simulink model "DIMR_ordinary"  (R2024b)
settings: Solver=daessc  StartTime=0.0  StopTime=60  RelTol=1e-3
values from neighbouring files (symbols this model uses):
  d_m0 = d_mn    (= 0)    [DIMR_main.m]
  d_m_cmd = 0.12787808985686    (= 0.127878089857)    [DIMR_main.m]
  dis_cmd = 0    [DIMR_main.m]
  jrk_cmd = 0.15    [DIMR_main.m]
  phi_cmd = 0*pi/180    (= 0)    [DIMR_main.m]
  ta = (vel_cmd-jrk_cmd*tt^2)/acc_cmd    (= 3.66666666667)    [DIMR_main.m]
  taz = z_vel_cmd/z_acc_cmd    (= 1.6)    [DIMR_main.m]
  tc = (x_cmd-2*(1/2*acc_cmd*ta^2+1/2*jrk_cmd*tt^2*ta+tt*vel_cmd))/vel_cmd    (= 10.6666666667)    [DIMR_main.m]
  tcz = (z_cmd-z_acc_cmd*taz^2)/z_vel_cmd    [DIMR_main.m]
  tcz2 = (z_cmd2-z_acc_cmd*taz^2)/z_vel_cmd    (= 0.9)    [DIMR_main.m]
  theta_f0 = -theta_p0    (= -0.024)    [DIMR_main.m]
  theta_f_cmd = 0.037940459    [DIMR_main.m]
  theta_p0 = theta_pn    (= 0.024)    [DIMR_main.m]
  theta_p_cmd = -0.037940459    [DIMR_main.m]
  ts = 15    [DIMR_main.m]
  ts2 = te+5    (= 39.3333333333)    [DIMR_main.m]
  tsz = 10    [DIMR_main.m]
  tsz2 = ts2    (= 39.3333333333)    [DIMR_main.m]
  tt = acc_cmd/jrk_cmd    (= 0.333333333333)    [DIMR_main.m]
  x_cmd = 3    [DIMR_main.m]
  z_0 = R_wo+L_bmy+L_my/2    [DIMR_main.m]
  z_acc_cmd = 0.05    [DIMR_main.m]
  z_cmd = 0.9-z_0    [DIMR_main.m]
  z_cmd2 = 0.9-0.7    (= 0.2)    [DIMR_main.m]
undefined symbols (not defined in the file or in its folder): Ac, Dc, DiscIntNeverNeededParam, dspblkCoreblockFVToolHelper, g, g_ext, g_fork, g_lift, g_reac, g_spado, g_yaw, gcbh, K_fd, K_fp, K_md, K_mp, K_pd, K_pp, K_wd, K_wi, K_wp, K_yd, K_yp, Kc, L_bg, L_bmx, L_bmy, L_bmz, L_bsx, L_bsy, L_bsz, L_by, L_ex, L_ey, L_ez, L_fg, L_fh, L_fx, L_fy, L_fz, L_lx, L_ly, L_lz, L_mg, L_mx, L_my, L_mz, L_wt, M_b, M_f, M_m, M_n11, M_n21, M_n22, M_n33, M_n44, Mc, N_f, N_w, omega_c ... (+10)
libraries: simulink x56, sm_lib x54, nesl_utility x12, slctrl_autotuning x1, slpidlib x1
(part 4 of 6)

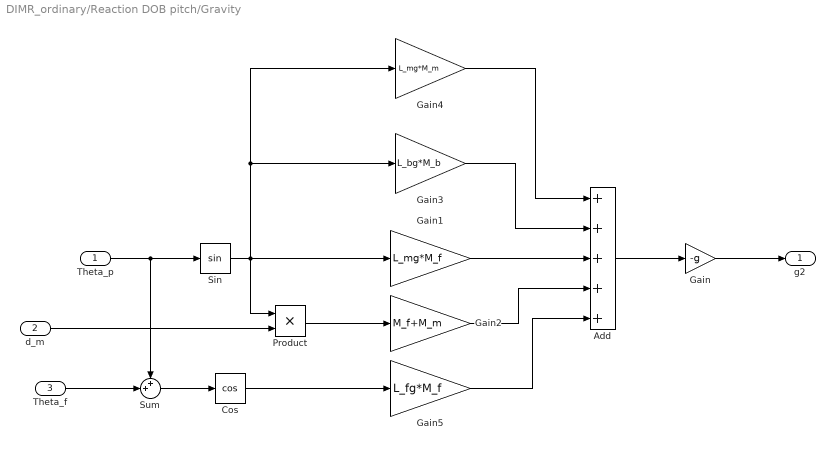
== system DIMR_ordinary/Reaction DOB pitch/Gravity ==
  Theta_p : Inport
  d_m : Inport  Port=2
  Theta_f : Inport  Port=3
  Add : Sum  Inputs=+++++
  Cos : Trigonometry  Operator=cos
  Gain : Gain  Gain=-g
  Gain1 : Gain  Gain=L_mg*M_f
  Gain2 : Gain  Gain=M_f+M_m
  Gain3 : Gain  Gain=L_bg*M_b
  Gain4 : Gain  Gain=L_mg*M_m
  Gain5 : Gain  Gain=L_fg*M_f
  Product : Product
  Sin : Trigonometry
  Sum : Sum  Inputs=++|
  g2 : Outport
  wires:
  Gain/1 -> g2/1
  Theta_p/1 -> Sin/1, Sum/1
  Sin/1 -> Gain4/1, Gain3/1, Product/1, Gain1/1
  d_m/1 -> Product/2
  Product/1 -> Gain2/1
  Theta_f/1 -> Sum/2
  Sum/1 -> Cos/1
  Cos/1 -> Gain5/1
  Add/1 -> Gain/1
  Gain4/1 -> Add/1
  Gain3/1 -> Add/2
  Gain1/1 -> Add/3
  Gain2/1 -> Add/4
  Gain5/1 -> Add/5

== matlab function DIMR_ordinary/IK1 ==
  data: dz input; tau input; z input; ik_theta1 output; ik_delta2 output; ik_dtheta1 output; ik_ddelta2 output; ik_lt output
function [ik_theta1,ik_delta2,ik_dtheta1,ik_ddelta2,ik_lt] = IK1(dz,tau,z)
%#codegen

%    This function was generated by the Symbolic Math Toolbox version 24.2.
%    15-Apr-2025 18:25:07

% dz = complex(dz);  % if required to enforce complex operations
% tau = complex(tau);  % if required to enforce complex operations
% z = complex(z);  % if required to enforce complex operations
t0 = roots([1.0,(tau.*8.44424930131968e+16-z.*6.07271847679102e+19-tau.*z.*1.125899906842624e+18+2.195986091984785e+19)./(tau.*1.238489897526886e+17+9.351986454258171e+17),0.0,((tau.*-8.44424930131968e+16+z.*6.07271847679102e+19+tau.*z.*1.125899906842624e+18+1.285078320466132e+19).*(-1.0./4.4e+2))./(tau.*2.81474976710656e+14+2.125451466876857e+15),-1.0]);
t2 = real(t0(4));
t3 = atan2(t2,1);
t4 = t2.^2;
t5 = t2.^3;
t6 = tau.^2;
t7 = tau.^3;
t9 = tau.^5;
t11 = z.^2;
t12 = z.^3;
t14 = z.^5;
t19 = tau.*1.40737488355328e+14;
t20 = tau.*5.319877059831398e+17;
t21 = t2.*tau.*1.238489897526886e+17;
t22 = t2.*9.351986454258171e+17;
t23 = tau.*z.*1.125899906842624e+18;
t24 = z.*6.07271847679102e+19;
t35 = tau.*4.635073695354219e-1;
t57 = tau.*5.743900035854321e+113;
t66 = tau.*z.*7.990597029423474e+114;
t74 = z.*1.447317376015955e+116;
t8 = t6.^2;
t10 = t6.^3;
t13 = t11.^2;
t15 = t11.^3;
t16 = t3.*2.0;
ik_theta1 = t16;
if nargout > 1
    t25 = -t23;
    t26 = -t24;
    t27 = t4.*tau.*8.44424930131968e+16;
    t28 = t5.*tau.*1.238489897526886e+17;
    t29 = t5.*9.351986454258171e+17;
    t30 = t4.*2.195986091984785e+19;
    t33 = t4.*tau.*z.*-1.125899906842624e+18;
    t34 = t4.*z.*-6.07271847679102e+19;
    t36 = t19+7.590898095988775e+15;
    t38 = t35+7.0./2.0;
    t39 = t35+6.81e+2./1.0e+1;
    t42 = t9.*2.386050182016105e+106;
    t46 = t9.*z.*4.211088297564564e+107;
    t51 = t7.*2.507343178421252e+110;
    t52 = t9.*t11.*4.593987726794744e+108;
    t58 = t9.*t12.*2.604615627247899e+109;
    t60 = t6.*2.999842761429269e+112;
    t61 = t7.*z.*9.409126505705104e+111;
    t65 = t9.*t14.*2.966510080312107e+110;
    t72 = -t66;
    t73 = t6.*z.*3.660741181676567e+113;
    t75 = t7.*t11.*6.407841099867219e+112;
    t76 = t7.*t12.*3.958710038416369e+112;
    t81 = -t74;
    t86 = t11.*tau.*3.585353509436109e+115;
    t87 = t6.*t11.*2.09113906624741e+114;
    t88 = t6.*t12.*3.785302651403782e+114;
    t90 = t7.*t14.*2.876678343420641e+114;
    t92 = t11.*7.09032593341523e+116;
    t93 = t12.*tau.*2.133985804221304e+116;
    t95 = t12.*3.242008287042286e+117;
    t98 = t14.*2.256895254686051e+118;
    t101 = t14.*tau.*2.510610198759619e+117;
    t102 = t6.*t14.*1.163686329155874e+116;
    t17 = cos(t16);
    t18 = sin(t16);
    t37 = 1.0./t36;
    t40 = 1.0./t39.^2;
    t41 = t10.*3.212055390272792e+104;
    t43 = t10.*z.*2.675474179773727e+105;
    t44 = t8.*2.477746168797788e+107;
    t47 = t10.*t11.*2.526492816377412e+106;
    t48 = -t46;
    t49 = t10.*t12.*1.059207781794524e+107;
    t50 = t10.*t13.*4.676525342669896e+107;
    t54 = t10.*t14.*9.166661893505187e+107;
    t55 = t10.*t15.*2.037035976334486e+108;
    t56 = t8.*z.*9.736596647488009e+109;
    t63 = -t58;
    t64 = t9.*t13.*1.239018969121646e+110;
    t67 = -t61;
    t68 = t8.*t11.*7.882227863274746e+110;
    t69 = t8.*t12.*2.154890938178742e+111;
    t70 = -t65;
    t71 = t9.*t15.*6.592244622915794e+110;
    t78 = t8.*t13.*1.21830758387732e+112;
    t79 = t8.*t14.*4.00008483587525e+112;
    t80 = -t73;
    t82 = -t76;
    t83 = t7.*t13.*4.915417942081258e+113;
    t85 = t8.*t15.*8.88907741305611e+112;
    t89 = t6.*t13.*1.928403609769147e+114;
    t91 = t7.*t15.*6.392618540934758e+114;
    t94 = t13.*tau.*3.97502326562149e+116;
    t96 = -t90;
    t97 = t13.*7.985575221783389e+117;
    t99 = t15.*5.015322788191225e+118;
    t103 = t6.*t15.*2.585969620346386e+116;
    t105 = -t98;
    t106 = -t101;
    t107 = t15.*tau.*5.579133775021375e+117;
    t108 = -t102;
    t109 = t20+t21+t22+t25+t26+t27+t28+t29+t30+t33+t34+2.869359480283757e+19;
    t45 = -t43;
    t53 = -t49;
    t59 = -t54;
    t62 = -t56;
    t77 = -t69;
    t84 = -t79;
    t100 = -t94;
    t104 = -t97;
    t110 = (t37.*t109)./8.0e+3;
    ik_delta2 = -t110;
end
if nargout > 2
    t111 = t110-1.59e+2./4.0e+2;
    t112 = t41+t42+t44+t45+t47+t48+t50+t51+t52+t53+t55+t57+t59+t60+t62+t63+t64+t67+t68+t70+t71+t72+t75+t77+t78+t80+t81+t82+t83+t84+t85+t86+t87+t88+t89+t91+t92+t93+t95+t96+t99+t100+t103+t104+t105+t106+t107+t108-2.105477541297374e+115;
    t113 = 1.0./t112;
    et1 = t2.*-1.753894605876528e+96+t4.*1.009464978528226e+96;
    et2 = t5.*4.619988807297373e+94-t6.*2.554852704393891e+92;
    et3 = t7.*-7.8111064788263e+89-t8.*1.00794759003273e+89;
    et4 = t9.*1.814387972119789e+86+t11.*6.245124509053326e+96;
    et5 = t12.*-3.331857083120826e+97;
    et6 = t13.*3.815554989087441e+97-tau.*5.24829876676123e+94;
    et7 = z.*1.399328629129073e+96-t2.*t6.*1.075720720231548e+91;
    et8 = t2.*t7.*-1.388092428471541e+90+t2.*t8.*7.128076116355089e+88;
    et9 = t4.*t6.*1.722969069981006e+93+t2.*t9.*1.361707336651519e+86;
    et10 = t4.*t7.*-1.973567476521639e+90+t5.*t6.*9.078257330103773e+92;
    et11 = t4.*t8.*1.151036106739522e+89+t5.*t7.*6.111449310419045e+90;
    et12 = t2.*t11.*5.875732481208788e+97+t4.*t9.*1.343184695804828e+87;
    et13 = t5.*t8.*-2.551325158332646e+88-t2.*t12.*1.782863198738202e+97;
    et14 = t5.*t9.*5.322204718218049e+86-t2.*t13.*5.464130766461227e+98;
    et15 = t4.*t11.*4.415911382468272e+97;
    et16 = t2.*t14.*8.258777032656798e+98;
    et17 = t4.*t12.*-8.469349253727501e+97;
    et18 = t5.*t11.*9.380726613532944e+95;
    et19 = t4.*t13.*6.359258315145734e+97;
    et20 = t5.*t12.*-1.175190936638932e+96+t6.*t11.*5.907708747848193e+94;
    et21 = t6.*t12.*-3.196898258866477e+95+t7.*t11.*1.247609721739556e+93;
    et22 = t6.*t13.*4.534279766579717e+95-t7.*t12.*6.544610701214467e+93;
    et23 = t8.*t11.*1.242487226117768e+91+t7.*t13.*1.139418916775499e+94;
    et24 = t8.*t12.*-5.845583673798496e+91+t9.*t11.*4.904790067467224e+88;
    et25 = t8.*t13.*1.333203858988986e+92-t9.*t12.*1.791158880389735e+89;
    et26 = t9.*t13.*5.970529601299116e+89+tau.*t2.*1.323988270291723e+93;
    et27 = t4.*tau.*1.468522013529346e+95+t5.*tau.*1.261219729665987e+94;
    et28 = t11.*tau.*1.207196483550789e+96;
    et29 = t12.*tau.*-6.477833809662083e+96;
    et30 = t13.*tau.*7.882625873837409e+96;
    et31 = z.*t2.*-1.890970205684437e+96;
    et32 = t4.*z.*-1.069218722198518e+97;
    et33 = t5.*z.*-3.150739272925472e+95+t6.*z.*2.668557352126731e+93;
    et34 = t7.*z.*4.092978643690637e+91+t8.*z.*6.846342443053817e+89;
    et35 = t9.*z.*-5.342131360762384e+87+tau.*z.*2.034429880145039e+95;
    et36 = t2.*t6.*t11.*3.834597488658114e+94+t2.*t6.*t12.*1.79267290146031e+95;
    et37 = t2.*t7.*t11.*3.241447763154754e+92-t2.*t6.*t13.*1.552786419763549e+96;
    et38 = t2.*t7.*t12.*4.397794916127146e+93+t2.*t8.*t11.*6.696326945473049e+89;
    et39 = t4.*t6.*t11.*2.979273638991897e+95;
    et40 = t2.*t6.*t14.*2.838892916716577e+96;
    et41 = t2.*t7.*t13.*-2.577198424443163e+94+t2.*t8.*t12.*4.358240682659937e+91;
    et42 = t2.*t9.*t11.*-1.748415316198616e+88-t4.*t6.*t12.*7.776982869967544e+95;
    et43 = t4.*t7.*t11.*4.360273950273173e+93+t5.*t6.*t11.*2.746751487155486e+94;
    et44 = t2.*t7.*t14.*5.263391152880169e+94-t2.*t8.*t13.*2.109408183024797e+92;
    et45 = t2.*t9.*t12.*1.455542746740951e+89+t4.*t6.*t13.*7.557132944299528e+95;
    et46 = t4.*t7.*t12.*-1.507615643654141e+94+t4.*t8.*t11.*2.876061807193666e+91;
    et47 = t5.*t6.*t12.*-3.913495645809803e+94+t5.*t7.*t11.*8.312588465463616e+92;
    et48 = t2.*t8.*t14.*4.879241176214998e+92-t2.*t9.*t13.*6.784692728748996e+89;
    et49 = t4.*t7.*t13.*1.899031527959165e+94-t4.*t8.*t12.*1.220393558543954e+92;
    et50 = t4.*t9.*t11.*1.010114099713122e+89-t5.*t7.*t12.*1.474838834239447e+93;
    et51 = t5.*t8.*t11.*9.289616355673145e+90+t2.*t9.*t14.*1.809251394333066e+90;
    et52 = t4.*t8.*t13.*2.22200643164831e+92-t4.*t9.*t12.*2.985264800649558e+89;
    et53 = t5.*t8.*t12.*-2.32376788561945e+91+t5.*t9.*t11.*2.955412152643063e+88;
    et54 = t4.*t9.*t13.*9.950882668831861e+89-t5.*t9.*t12.*1.313516512285806e+89;
    et55 = t2.*t11.*tau.*2.467684994491885e+96;
    et56 = t2.*t12.*tau.*2.151307797149133e+96;
    et57 = t2.*t13.*tau.*-4.626464408073966e+97;
    et58 = t4.*t11.*tau.*7.861141246672502e+96;
    et59 = t2.*t14.*tau.*7.65600803597262e+97;
    et60 = t4.*t12.*tau.*-1.628045107945128e+97;
    et61 = t5.*t11.*tau.*2.881458695288517e+95;
    et62 = t4.*t13.*tau.*1.313770978972902e+97;
    et63 = t5.*t12.*tau.*-3.766278218797084e+95-t2.*t6.*z.*8.69453683410162e+92;
    et64 = t2.*t7.*z.*-8.14011166039339e+90-t2.*t8.*z.*7.354331859382801e+89;
    et65 = t4.*t6.*z.*-4.607531607862968e+94-t2.*t9.*z.*1.094057710499569e+87;
    et66 = t4.*t7.*z.*-4.316771097086506e+92-t5.*t6.*z.*7.922329257005371e+93;
    et67 = t4.*t8.*z.*-2.629642166088229e+90-t5.*t7.*z.*1.751142096260925e+92;
    et68 = t4.*t9.*z.*-1.179328859496608e+88-t5.*t8.*z.*1.536226654469186e+90;
    et69 = t5.*t9.*z.*-8.573979033945596e+87-tau.*z.*t2.*1.644111357410597e+95;
    et70 = t4.*tau.*z.*-1.740373755123545e+96;
    et71 = t5.*tau.*z.*-9.219656825165702e+94-3.817418975922806e+95;
    ik_dtheta1 = dz.*t36.*t113.*(et1+et2+et3+et4+et5+et6+et7+et8+et9+et10+et11+et12+et13+et14+et15+et16+et17+et18+et19+et20+et21+et22+et23+et24+et25+et26+et27+et28+et29+et30+et31+et32+et33+et34+et35+et36+et37+et38+et39+et40+et41+et42+et43+et44+et45+et46+et47+et48+et49+et50+et51+et52+et53+et54+et55+et56+et57+et58+et59+et60+et61+et62+et63+et64+et65+et66+et67+et68+et69+et70+et71).*8.0e+3;
end
if nargout > 3
    et72 = t2.*-3.7071702195569e+114;
    et73 = t4.*3.804188113277026e+115;
    et74 = t5.*1.625202646823668e+114;
    et75 = t6.*1.140152959101139e+112;
    et76 = t7.*3.851536071140141e+109;
    et77 = t8.*4.771323709725432e+107;
    et78 = t9.*2.37036597763644e+105;
    et79 = t10.*3.344342724717159e+103;
    et80 = t11.*6.661710042517029e+116;
    et81 = t12.*3.317645224682185e+117;
    et82 = t13.*-8.033152579881287e+117+t55+t59+t70+t71+t84+t85+t91+t96+t99+t103+t105+t106+t107+t108;
    et83 = tau.*3.305389407105682e+113;
    et84 = z.*-1.344576683503948e+116;
    et85 = t2.*t6.*-5.521484071666565e+111;
    et86 = t2.*t7.*-1.201004210046715e+109;
    et87 = t2.*t8.*-1.446897405085628e+108;
    et88 = t4.*t6.*-7.600317735708989e+111;
    et89 = t2.*t9.*-6.836757611015585e+105;
    et90 = t4.*t7.*9.237917051294251e+109;
    et91 = t5.*t6.*-8.407795288014511e+110;
    et92 = t2.*t10.*4.905035996251834e+103;
    et93 = t4.*t8.*6.21766718480593e+107;
    et94 = t5.*t7.*-1.679675237605966e+109;
    et95 = t2.*t11.*2.425689270038724e+115;
    et96 = t4.*t9.*-2.369824972154481e+105;
    et97 = t5.*t8.*1.018828318361818e+108;
    et98 = t2.*t12.*-6.307571438901966e+116;
    et99 = t4.*t10.*3.344342724717159e+103;
    et100 = t5.*t9.*7.067802508371117e+105;
    et101 = t2.*t13.*1.396484281539863e+117;
    et102 = t4.*t11.*-1.402659673535802e+117;
    et103 = t5.*t10.*4.905035996251834e+103;
    et104 = t2.*t14.*-7.723597093814486e+116;
    et105 = t4.*t12.*3.938271388021781e+117;
    et106 = t5.*t11.*-5.533248821789028e+115;
    et107 = t4.*t13.*1.098783857622504e+118;
    et108 = t5.*t12.*1.557427551233363e+115;
    et109 = t6.*t11.*7.991271506884402e+113;
    et110 = t4.*t14.*-5.131828736560907e+118;
    et111 = t5.*t13.*5.110047691224071e+116;
    et112 = t6.*t12.*6.388892406797049e+114;
    et113 = t7.*t11.*2.225465716458933e+112;
    et114 = t5.*t14.*-7.723597093814486e+116;
    et115 = t6.*t13.*6.133630224665161e+112;
    et116 = t7.*t12.*6.414800515945154e+112;
    et117 = t8.*t11.*2.190420013370623e+110;
    et118 = t7.*t13.*4.024585580613185e+113;
    et119 = t8.*t12.*-3.271771400537028e+110;
    et120 = t9.*t11.*9.648630921792687e+107;
    et121 = t8.*t13.*1.013528935640283e+112;
    et122 = t9.*t12.*-1.235951960272058e+109;
    et123 = t10.*t11.*1.239367190298751e+106;
    et124 = t9.*t13.*1.011419526100604e+110;
    et125 = t10.*t12.*-7.63430158030757e+106;
    et126 = t10.*t13.*3.690599930124005e+107+t4.*t55+t4.*t71+t4.*t85+t4.*t91+t4.*t99+t4.*t103+t4.*t107;
    et127 = tau.*t2.*-5.325511928164662e+113;
    et128 = t4.*tau.*-4.601389533003556e+111;
    et129 = t5.*tau.*2.102524928619955e+113;
    et130 = t11.*tau.*2.257239068666816e+115;
    et131 = t12.*tau.*2.379035049732175e+116;
    et132 = t13.*tau.*-4.136321230248881e+116;
    et133 = z.*t2.*3.113201852556033e+115;
    et134 = t4.*z.*-6.511422436340579e+115;
    et135 = t5.*z.*1.662776353932113e+114;
    et136 = t6.*z.*-9.989623857325219e+112;
    et137 = t7.*z.*-3.096673052545432e+111;
    et138 = t8.*z.*-3.937587938067827e+109;
    et139 = t9.*z.*-6.92947223565074e+106;
    et140 = t10.*z.*-1.077535567389974e+105;
    et141 = tau.*z.*-4.956122630630957e+114;
    et142 = t2.*t6.*t11.*5.463288101128978e+113;
    et143 = t2.*t6.*t12.*-6.870842133918736e+114;
    et144 = t2.*t7.*t11.*1.493465513298907e+112;
    et145 = t2.*t6.*t13.*1.770473980809039e+115;
    et146 = t2.*t7.*t12.*-1.662839869670821e+113;
    et147 = t2.*t8.*t11.*1.600464698420783e+110;
    et148 = t4.*t6.*t11.*-1.185362385403583e+114;
    et149 = t2.*t6.*t14.*-1.213681741815904e+115;
    et150 = t2.*t7.*t13.*4.808389969487753e+113;
    et151 = t2.*t8.*t12.*-2.039300901034873e+111;
    et152 = t2.*t9.*t11.*9.085779705955538e+107;
    et153 = t4.*t6.*t12.*1.484825663584366e+113;
    et154 = t4.*t7.*t11.*-6.414166966086719e+111;
    et155 = t5.*t6.*t11.*-3.653957848263659e+113;
    et156 = t2.*t7.*t14.*-4.008171825166093e+113;
    et157 = t2.*t8.*t13.*6.483084785515751e+111;
    et158 = t2.*t9.*t12.*-1.26913217775301e+109;
    et159 = t2.*t10.*t11.*5.825642799869884e+105;
    et160 = t4.*t6.*t13.*5.411483176200627e+115;
    et161 = t4.*t7.*t12.*-8.894206859842618e+112;
    et162 = t4.*t8.*t11.*5.436080491457138e+109;
    et163 = t5.*t6.*t12.*-5.173317577586963e+113;
    et164 = t5.*t7.*t11.*-6.429724676055676e+111;
    et165 = t2.*t8.*t14.*-6.974962743444695e+111;
    et166 = t2.*t9.*t13.*4.061517620170128e+109;
    et167 = t2.*t10.*t12.*-3.429451917957924e+106;
    et168 = t4.*t6.*t14.*-2.15192323946998e+116;
    et169 = t4.*t7.*t13.*1.299597929976685e+114;
    et170 = t4.*t8.*t12.*-1.844308794184032e+111;
    et171 = t4.*t9.*t11.*1.573497725719581e+108;
    et172 = t5.*t6.*t13.*7.181993187065789e+114;
    et173 = t5.*t7.*t12.*-3.254097673006372e+112;
    et174 = t5.*t8.*t11.*-6.043433221327569e+109;
    et175 = t2.*t9.*t14.*-6.212091849660983e+109;
    et176 = t2.*t10.*t13.*8.402773402379755e+106;
    et177 = t4.*t7.*t14.*-4.708898706530657e+114;
    et178 = t4.*t8.*t13.*1.74782751136632e+112;
    et179 = t4.*t9.*t12.*-1.742635765920156e+109;
    et180 = t4.*t10.*t11.*1.239367190298751e+106;
    et181 = t5.*t6.*t14.*-1.213681741815904e+115;
    et182 = t5.*t7.*t13.*2.164129541447379e+113;
    et183 = t5.*t8.*t12.*-7.898098107882316e+110;
    et184 = t5.*t9.*t11.*1.056305699482443e+107;
    et185 = t2.*t10.*t14.*-2.240739573967935e+107;
    et186 = t4.*t8.*t14.*-5.698580117703968e+112;
    et187 = t4.*t9.*t13.*1.247599050175231e+110;
    et188 = t4.*t10.*t12.*-7.63430158030757e+106;
    et189 = t5.*t7.*t14.*-4.008171825166093e+113;
    et190 = t5.*t8.*t13.*3.389105780136559e+111;
    et191 = t5.*t9.*t12.*-8.534562153816679e+108;
    et192 = t5.*t10.*t11.*5.825642799869884e+105;
    et193 = t4.*t9.*t14.*-3.596322144511111e+110;
    et194 = t4.*t10.*t13.*3.690599930124005e+107;
    et195 = t5.*t8.*t14.*-6.974962743444695e+111;
    et196 = t5.*t9.*t13.*2.67593107893232e+109;
    et197 = t5.*t10.*t12.*-3.429451917957924e+106;
    et198 = t4.*t10.*t14.*-9.166661893505187e+107;
    et199 = t5.*t9.*t14.*-6.212091849660983e+109;
    et200 = t5.*t10.*t13.*8.402773402379755e+106;
    et201 = t5.*t10.*t14.*-2.240739573967935e+107;
    et202 = t2.*t11.*tau.*6.55228474510829e+114;
    et203 = t2.*t12.*tau.*-1.267703580425692e+116;
    et204 = t2.*t13.*tau.*2.938721960462308e+116;
    et205 = t4.*t11.*tau.*-7.04099589462565e+115;
    et206 = t2.*t14.*tau.*-1.738830026548328e+116;
    et207 = t4.*t12.*tau.*1.630150948443772e+116;
    et208 = t5.*t11.*tau.*-9.746468343421371e+114;
    et209 = t4.*t13.*tau.*1.19686993761682e+117;
    et210 = t5.*t12.*tau.*-3.016101165989628e+113;
    et211 = t4.*t14.*tau.*-5.175715910305871e+117;
    et212 = t5.*t13.*tau.*1.10939340005696e+116;
    et213 = t5.*t14.*tau.*-1.738830026548328e+116;
    et214 = t2.*t6.*z.*8.794648178204421e+112;
    et215 = t2.*t7.*z.*7.919641221873595e+110;
    et216 = t2.*t8.*z.*1.21602593543738e+109;
    et217 = t4.*t6.*z.*2.781622178886485e+112;
    et218 = t2.*t9.*z.*-2.896086435720579e+106;
    et219 = t4.*t7.*z.*-2.055401707707991e+110;
    et220 = t5.*t6.*z.*1.514114329663636e+112;
    et221 = t2.*t10.*z.*-9.263806993383842e+104;
    et222 = t4.*t8.*z.*7.430651182143457e+108;
    et223 = t5.*t7.*z.*-1.961418471770079e+110;
    et224 = t4.*t9.*z.*-3.120986874463163e+106;
    et225 = t5.*t8.*z.*-1.733280133320865e+108;
    et226 = t4.*t10.*z.*-1.077535567389974e+105;
    et227 = t5.*t9.*z.*4.471769997311462e+106;
    et228 = t5.*t10.*z.*-9.263806993383842e+104;
    et229 = tau.*z.*t2.*4.747078578574793e+114;
    et230 = t4.*tau.*z.*1.829231727498887e+114;
    et231 = t5.*tau.*z.*3.448046785767965e+113;
    et232 = -2.19283328574275e+115;
    ik_ddelta2 = dz.*t113.*(et72+et73+et74+et75+et76+et77+et78+et79+et80+et81+et82+et83+et84+et85+et86+et87+et88+et89+et90+et91+et92+et93+et94+et95+et96+et97+et98+et99+et100+et101+et102+et103+et104+et105+et106+et107+et108+et109+et110+et111+et112+et113+et114+et115+et116+et117+et118+et119+et120+et121+et122+et123+et124+et125+et126+et127+et128+et129+et130+et131+et132+et133+et134+et135+et136+et137+et138+et139+et140+et141+et142+et143+et144+et145+et146+et147+et148+et149+et150+et151+et152+et153+et154+et155+et156+et157+et158+et159+et160+et161+et162+et163+et164+et165+et166+et167+et168+et169+et170+et171+et172+et173+et174+et175+et176+et177+et178+et179+et180+et181+et182+et183+et184+et185+et186+et187+et188+et189+et190+et191+et192+et193+et194+et195+et196+et197+et198+et199+et200+et201+et202+et203+et204+et205+et206+et207+et208+et209+et210+et211+et212+et213+et214+et215+et216+et217+et218+et219+et220+et221+et222+et223+et224+et225+et226+et227+et228+et229+et230+et231+et232);
end
if nargout > 4
    ik_lt = sqrt(t40.*(t17.*7.165375-t17.*t111.*(4.3e+1./2.0)+t38.*(t17.*(1.59e+2./4.0e+2)-(t17.*t37.*t109)./8.0e+3)).^2+t40.*(t18.*7.165375-t18.*t111.*(4.3e+1./2.0)+t38.*(t18.*(1.59e+2./4.0e+2)-(t18.*t37.*t109)./8.0e+3+1.1e+1./5.0e+1)).^2);
end
end

== matlab function DIMR_ordinary/Calc_states/MATLAB Function ==
  data: theta1 input; z output; delta2 input; theta3 input; r input; d2 input; dt input
function z = fcn(theta1, delta2, theta3, r, d2, dt)

z = r+cos(theta1)*(delta2+d2)-dt*sin(theta1*theta3);

== matlab function DIMR_ordinary/simp_model1 ==
  data: inv_cog_theta1 output; lt input; tau input; tau_w input; inv_cog_delta2 output; inv_cog_dtheta1 output; inv_cog_ddelta2 output
function [inv_cog_theta1,inv_cog_delta2,inv_cog_dtheta1,inv_cog_ddelta2] = simp_model1(lt,tau,tau_w)
%#codegen

%    This function was generated by the Symbolic Math Toolbox version 24.2.
%    15-Apr-2025 18:25:12

% lt = complex(lt);  % if required to enforce complex operations
% tau = complex(tau);  % if required to enforce complex operations
% tau_w = complex(tau_w);  % if required to enforce complex operations
t0 = roots([tau.*-1.447792593175879e+32-tau.*tan(atan(((lt.*3.671450002392298e+16-sqrt(lt.^2.*1.34795451200664e+33-tau_w.^2.*3.022314549036573e+27+lt.^2.*tau_w.^2.*4.75626088156714e+29)).*4.447070890666667e+5)./(tau_w.*2.444803076916086e+19-lt.*tau_w.*3.066951346239308e+20)).*2.0).^2.*1.447792593175879e+32-tan(atan(((lt.*3.671450002392298e+16-sqrt(lt.^2.*1.34795451200664e+33-tau_w.^2.*3.022314549036573e+27+lt.^2.*tau_w.^2.*4.75626088156714e+29)).*4.447070890666667e+5)./(tau_w.*2.444803076916086e+19-lt.*tau_w.*3.066951346239308e+20)).*2.0).^2.*5.46622816503927e+32+lt.^2.*tan(atan(((lt.*3.671450002392298e+16-sqrt(lt.^2.*1.34795451200664e+33-tau_w.^2.*3.022314549036573e+27+lt.^2.*tau_w.^2.*4.75626088156714e+29)).*4.447070890666667e+5)./(tau_w.*2.444803076916086e+19-lt.*tau_w.*3.066951346239308e+20)).*2.0).^2.*4.275634069905172e+36-tau.^2.*tan(atan(((lt.*3.671450002392298e+16-sqrt(lt.^2.*1.34795451200664e+33-tau_w.^2.*3.022314549036573e+27+lt.^2.*tau_w.^2.*4.75626088156714e+29)).*4.447070890666667e+5)./(tau_w.*2.444803076916086e+19-lt.*tau_w.*3.066951346239308e+20)).*2.0).^2.*9.586607664225985e+30-tau.^2.*9.586607664225985e+30+lt.^2.*tau.*tan(atan(((lt.*3.671450002392298e+16-sqrt(lt.^2.*1.34795451200664e+33-tau_w.^2.*3.022314549036573e+27+lt.^2.*tau_w.^2.*4.75626088156714e+29)).*4.447070890666667e+5)./(tau_w.*2.444803076916086e+19-lt.*tau_w.*3.066951346239308e+20)).*2.0).^2.*5.820228783664543e+34+lt.^2.*tau.^2.*tan(atan(((lt.*3.671450002392298e+16-sqrt(lt.^2.*1.34795451200664e+33-tau_w.^2.*3.022314549036573e+27+lt.^2.*tau_w.^2.*4.75626088156714e+29)).*4.447070890666667e+5)./(tau_w.*2.444803076916086e+19-lt.*tau_w.*3.066951346239308e+20)).*2.0).^2.*1.980704062856608e+32-5.46622816503927e+32,lt.^2.*tan(atan(((lt.*3.671450002392298e+16-sqrt(lt.^2.*1.34795451200664e+33-tau_w.^2.*3.022314549036573e+27+lt.^2.*tau_w.^2.*4.75626088156714e+29)).*4.447070890666667e+5)./(tau_w.*2.444803076916086e+19-lt.*tau_w.*3.066951346239308e+20)).*2.0).*1.710253627962069e+37+lt.^2.*tau.^2.*tan(atan(((lt.*3.671450002392298e+16-sqrt(lt.^2.*1.34795451200664e+33-tau_w.^2.*3.022314549036573e+27+lt.^2.*tau_w.^2.*4.75626088156714e+29)).*4.447070890666667e+5)./(tau_w.*2.444803076916086e+19-lt.*tau_w.*3.066951346239308e+20)).*2.0).*7.922816251426434e+32+lt.^2.*tau.*tan(atan(((lt.*3.671450002392298e+16-sqrt(lt.^2.*1.34795451200664e+33-tau_w.^2.*3.022314549036573e+27+lt.^2.*tau_w.^2.*4.75626088156714e+29)).*4.447070890666667e+5)./(tau_w.*2.444803076916086e+19-lt.*tau_w.*3.066951346239308e+20)).*2.0).*2.328091513465817e+35,tau.*2.895585186351758e+32+tau.*tan(atan(((lt.*3.671450002392298e+16-sqrt(lt.^2.*1.34795451200664e+33-tau_w.^2.*3.022314549036573e+27+lt.^2.*tau_w.^2.*4.75626088156714e+29)).*4.447070890666667e+5)./(tau_w.*2.444803076916086e+19-lt.*tau_w.*3.066951346239308e+20)).*2.0).^2.*2.895585186351758e+32+tan(atan(((lt.*3.671450002392298e+16-sqrt(lt.^2.*1.34795451200664e+33-tau_w.^2.*3.022314549036573e+27+lt.^2.*tau_w.^2.*4.75626088156714e+29)).*4.447070890666667e+5)./(tau_w.*2.444803076916086e+19-lt.*tau_w.*3.066951346239308e+20)).*2.0).^2.*1.093245633007854e+33+lt.^2.*tau.*2.328091513465817e+35-lt.^2.*tan(atan(((lt.*3.671450002392298e+16-sqrt(lt.^2.*1.34795451200664e+33-tau_w.^2.*3.022314549036573e+27+lt.^2.*tau_w.^2.*4.75626088156714e+29)).*4.447070890666667e+5)./(tau_w.*2.444803076916086e+19-lt.*tau_w.*3.066951346239308e+20)).*2.0).^2.*8.551268139810345e+36+tau.^2.*tan(atan(((lt.*3.671450002392298e+16-sqrt(lt.^2.*1.34795451200664e+33-tau_w.^2.*3.022314549036573e+27+lt.^2.*tau_w.^2.*4.75626088156714e+29)).*4.447070890666667e+5)./(tau_w.*2.444803076916086e+19-lt.*tau_w.*3.066951346239308e+20)).*2.0).^2.*1.917321532845197e+31+lt.^2.*1.710253627962069e+37+tau.^2.*1.917321532845197e+31+lt.^2.*tau.^2.*7.922816251426434e+32-lt.^2.*tau.*tan(atan(((lt.*3.671450002392298e+16-sqrt(lt.^2.*1.34795451200664e+33-tau_w.^2.*3.022314549036573e+27+lt.^2.*tau_w.^2.*4.75626088156714e+29)).*4.447070890666667e+5)./(tau_w.*2.444803076916086e+19-lt.*tau_w.*3.066951346239308e+20)).*2.0).^2.*1.164045756732909e+35-lt.^2.*tau.^2.*tan(atan(((lt.*3.671450002392298e+16-sqrt(lt.^2.*1.34795451200664e+33-tau_w.^2.*3.022314549036573e+27+lt.^2.*tau_w.^2.*4.75626088156714e+29)).*4.447070890666667e+5)./(tau_w.*2.444803076916086e+19-lt.*tau_w.*3.066951346239308e+20)).*2.0).^2.*3.961408125713217e+32+1.093245633007854e+33,lt.^2.*tan(atan(((lt.*3.671450002392298e+16-sqrt(lt.^2.*1.34795451200664e+33-tau_w.^2.*3.022314549036573e+27+lt.^2.*tau_w.^2.*4.75626088156714e+29)).*4.447070890666667e+5)./(tau_w.*2.444803076916086e+19-lt.*tau_w.*3.066951346239308e+20)).*2.0).*-1.710253627962069e+37-lt.^2.*tau.^2.*tan(atan(((lt.*3.671450002392298e+16-sqrt(lt.^2.*1.34795451200664e+33-tau_w.^2.*3.022314549036573e+27+lt.^2.*tau_w.^2.*4.75626088156714e+29)).*4.447070890666667e+5)./(tau_w.*2.444803076916086e+19-lt.*tau_w.*3.066951346239308e+20)).*2.0).*7.922816251426434e+32-lt.^2.*tau.*tan(atan(((lt.*3.671450002392298e+16-sqrt(lt.^2.*1.34795451200664e+33-tau_w.^2.*3.022314549036573e+27+lt.^2.*tau_w.^2.*4.75626088156714e+29)).*4.447070890666667e+5)./(tau_w.*2.444803076916086e+19-lt.*tau_w.*3.066951346239308e+20)).*2.0).*2.328091513465817e+35,tau.*-1.447792593175879e+32-tau.*tan(atan(((lt.*3.671450002392298e+16-sqrt(lt.^2.*1.34795451200664e+33-tau_w.^2.*3.022314549036573e+27+lt.^2.*tau_w.^2.*4.75626088156714e+29)).*4.447070890666667e+5)./(tau_w.*2.444803076916086e+19-lt.*tau_w.*3.066951346239308e+20)).*2.0).^2.*1.447792593175879e+32-tan(atan(((lt.*3.671450002392298e+16-sqrt(lt.^2.*1.34795451200664e+33-tau_w.^2.*3.022314549036573e+27+lt.^2.*tau_w.^2.*4.75626088156714e+29)).*4.447070890666667e+5)./(tau_w.*2.444803076916086e+19-lt.*tau_w.*3.066951346239308e+20)).*2.0).^2.*5.46622816503927e+32+lt.^2.*tan(atan(((lt.*3.671450002392298e+16-sqrt(lt.^2.*1.34795451200664e+33-tau_w.^2.*3.022314549036573e+27+lt.^2.*tau_w.^2.*4.75626088156714e+29)).*4.447070890666667e+5)./(tau_w.*2.444803076916086e+19-lt.*tau_w.*3.066951346239308e+20)).*2.0).^2.*4.275634069905172e+36-tau.^2.*tan(atan(((lt.*3.671450002392298e+16-sqrt(lt.^2.*1.34795451200664e+33-tau_w.^2.*3.022314549036573e+27+lt.^2.*tau_w.^2.*4.75626088156714e+29)).*4.447070890666667e+5)./(tau_w.*2.444803076916086e+19-lt.*tau_w.*3.066951346239308e+20)).*2.0).^2.*9.586607664225985e+30-tau.^2.*9.586607664225985e+30+lt.^2.*tau.*tan(atan(((lt.*3.671450002392298e+16-sqrt(lt.^2.*1.34795451200664e+33-tau_w.^2.*3.022314549036573e+27+lt.^2.*tau_w.^2.*4.75626088156714e+29)).*4.447070890666667e+5)./(tau_w.*2.444803076916086e+19-lt.*tau_w.*3.066951346239308e+20)).*2.0).^2.*5.820228783664543e+34+lt.^2.*tau.^2.*tan(atan(((lt.*3.671450002392298e+16-sqrt(lt.^2.*1.34795451200664e+33-tau_w.^2.*3.022314549036573e+27+lt.^2.*tau_w.^2.*4.75626088156714e+29)).*4.447070890666667e+5)./(tau_w.*2.444803076916086e+19-lt.*tau_w.*3.066951346239308e+20)).*2.0).^2.*1.980704062856608e+32-5.46622816503927e+32]);
if tau_w >= 0
    t2 = real(t0(4));
else
    t2 = real(t0(3));
end
inv_cog_theta1 = atan(t2).*2.0;
if nargout > 1
    t3 = lt.^2;
    t4 = tau.^2;
    t5 = tau_w.^2;
    t6 = tau_w.*4.0e+2;
    t7 = tau.*1.40737488355328e+14;
    t8 = tau.*2.81474976710656e+14;
    t9 = lt.*3.671450002392298e+16;
    t14 = tau.*1.447792593175879e+32;
    t22 = lt.*tau_w.*5.017911463213649e+3;
    t10 = t5.*3.022314549036573e+27;
    t12 = t8+2.125451466876857e+15;
    t13 = t7+7.590898095988775e+15;
    t15 = t4.*9.586607664225985e+30;
    t18 = t3.*1.34795451200664e+33;
    t19 = t3.*tau.*2.328091513465817e+35;
    t20 = t3.*t4.*7.922816251426434e+32;
    t21 = t3.*1.710253627962069e+37;
    t23 = -t22;
    t26 = t3.*t5.*4.75626088156714e+29;
    t11 = -t10;
    t16 = 1.0./t13;
    t17 = 1.0./t12;
    t24 = t6+t23;
    t25 = 1.0./t24;
    t27 = t11+t18+t26;
    t28 = sqrt(t27);
    t29 = -t28;
    t30 = t9+t29;
    t31 = (t25.*t30)./1.37438953472e+11;
    t32 = atan(t31);
    t33 = t32.*2.0;
    t34 = tan(t33);
    t35 = t34.^2;
    t36 = t34.^3;
    t37 = t35+1.0;
    t39 = t35.*5.46622816503927e+32;
    t40 = t14.*t35;
    t41 = t15.*t35;
    t42 = t3.*t35.*tau.*5.820228783664543e+34;
    t43 = t3.*t4.*t35.*1.980704062856608e+32;
    t45 = t3.*t35.*4.275634069905172e+36;
    t38 = 1.0./t37;
    t44 = -t42;
    t46 = -t43;
    t47 = -t45;
    et1 = t4.*1.385700562374483e+33+t34.*2.186491266015708e+34+t35.*9.713061509417766e+35+t36.*2.186491266015708e+34+tau.*1.390943230767213e+35;
    et2 = t3.*t34.*-3.420507255924138e+38+t4.*t34.*3.834643065690394e+32-t3.*t36.*1.710253627962069e+38+t4.*t35.*1.385700562374483e+33+t4.*t36.*3.834643065690394e+32;
    et3 = t34.*tau.*5.791170372703516e+33+t35.*tau.*1.390943230767213e+35+t36.*tau.*5.791170372703516e+33-t3.*t4.*t34.*1.584563250285287e+34-t3.*t4.*t36.*7.922816251426434e+33;
    et4 = t3.*t34.*tau.*-4.656183026931634e+36-t3.*t36.*tau.*2.328091513465817e+36+9.713061509417766e+35;
    et5 = t4.*2.875982299267795e+31+t19+t20+t21+t35.*1.639868449511781e+33+t42+t43+t45+tau.*4.343377779527637e+32+t4.*t35.*2.875982299267795e+31+t35.*tau.*4.343377779527637e+32;
    et6 = 1.639868449511781e+33;
    et7 = t16.*t17.*t38.*(et1+et2+et3+et4).*(-1.136363636363636e-5)-(t2.*t16.*t17.*t38.*(et5+et6))./2.2e+3+(t2.^3.*t16.*t17.*t38.*(t14+t15+t39+t40+t41+t44+t46+t47+5.46622816503927e+32))./2.2e+3;
    et8 = (t2.^2.*t16.*t17.*t34.*t38.*(t14+t15-t19-t20-t21+t39+t44+t46+t47+t4.*t35.*9.586607664225985e+30+t35.*tau.*1.447792593175879e+32+5.46622816503927e+32))./2.2e+3;
    inv_cog_delta2 = et7+et8;
end
if nargout > 2
    inv_cog_dtheta1 = 0.0;
end
if nargout > 3
    inv_cog_ddelta2 = 0.0;
end
end

== matlab function DIMR_ordinary/MATLAB Function ==
  data: thp input; tht output; dm input; ml input; tl input; L_mg parameter; g parameter; L_fg parameter; M_b parameter; L_bg parameter; M_m parameter; M_f parameter
function tht = fcn(thp, dm, ml, tl, L_mg, g, L_fg, M_b, L_bg, M_m, M_f)

CoGx = ml*(dm*sin(thp)+L_mg*sin(thp)+tl/(g*ml))+M_f*(L_fg+dm*sin(thp)+L_mg*sin(thp))+M_b*L_bg*sin(thp)+M_m*sin(thp)*(dm+L_mg);

CoGz = ((M_f+ml+M_m)*(dm+L_mg)+L_bg*M_b)*cos(thp);

tht = atan2(CoGx,CoGz);

== matlab function DIMR_ordinary/IK_simp ==
  data: dz input; ik_theta1 output; mass_l input; tau input; z input; ik_delta2 output; ik_dtheta1 output; ik_ddelta2 output; ik_lt output
function [ik_theta1,ik_delta2,ik_dtheta1,ik_ddelta2,ik_lt] = IK_simp(dz,mass_l,tau,z)
%#codegen

%    This function was generated by the Symbolic Math Toolbox version 24.2.
%    22-Apr-2025 19:32:21

% dz = complex(dz);  % if required to enforce complex operations
% mass_l = complex(mass_l);  % if required to enforce complex operations
% tau = complex(tau);  % if required to enforce complex operations
% z = complex(z);  % if required to enforce complex operations
t2 = mass_l.^2;
t3 = mass_l.^3;
t4 = tau.^2;
t5 = z.^2;
t6 = z.^3;
t7 = mass_l+6.81e+2./1.0e+1;
t8 = z-1.89e+2./4.0e+2;
t10 = mass_l.*3.312391896431465e+18;
t11 = tau.*4.503599627370496e+18;
t13 = mass_l.*z.*4.416522528575287e+19;
t14 = z.*1.104130632143822e+21;
t16 = mass_l.*tau.*1.837859027370372e+41;
t18 = tau.*4.59464756842593e+42;
t26 = tau.*z.*6.12619675790124e+43;
t28 = mass_l.*9.896058306351893e+43;
t30 = mass_l.*tau.*z.*2.450478703160496e+42;
t34 = mass_l.*z.*3.907436012123506e+44;
t36 = z.*3.298686102117298e+46;
t9 = 1.0./t7.^2;
t12 = -t10;
t15 = t11+3.400722347002971e+19;
t17 = t3.*6.583164045326904e+39;
t19 = t4.*3.042361440547751e+41;
t20 = -t16;
t22 = mass_l.*t4.*1.2169445762191e+40;
t23 = -t18;
t25 = t3.*z.*2.633265618130762e+41;
t27 = t2.*1.393096259451853e+42;
t31 = mass_l.*t4.*z.*1.622592768292134e+41;
t32 = -t28;
t33 = t4.*z.*4.056481920730334e+42;
t35 = t2.*z.*3.056606954005584e+43;
t38 = t3.*t5.*3.511020824174349e+42;
t39 = t2.*t5.*7.21105160271675e+43;
t40 = t3.*t6.*1.560453699633044e+43;
t42 = t6.*2.438208905676631e+47;
t43 = t5.*1.547884732724281e+47;
t44 = mass_l.*t6.*2.925850686811957e+46;
t45 = mass_l.*t5.*1.018868984668528e+46;
t46 = t2.*t6.*1.170340274724783e+45;
t21 = -t17;
t24 = -t19;
t29 = -t22;
t37 = -t35;
t41 = -t38;
t47 = t12+t13+t14+2.336506037211149e+20;
t48 = 1.0./t47;
t52 = t20+t21+t23+t24+t25+t26+t27+t29+t30+t31+t32+t33+t34+t36+t37+t39+t40+t41+t42+t43+t44+t45+t46+2.293175436578048e+45;
t49 = t15.*t48;
ik_theta1 = -t49;
if nargout > 1
    ik_delta2 = t8;
end
if nargout > 2
    t53 = 1.0./t52;
    ik_dtheta1 = dz.*t53.*(mass_l+2.5e+1).*(tau.*5.62949953421312e+16+4.250902933753714e+17).*(mass_l.*-6.0e+2+z.*2.0e+5+mass_l.*z.*8.0e+3+4.2323e+4).*3.53321802286023e+21;
end
if nargout > 3
    et1 = mass_l.*-3.2242253922e+12+t2.*4.570884e+10-t3.*2.16e+8+t5.*5.07876e+15+t6.*8.0e+15+z.*1.0747417974e+15+mass_l.*t5.*3.343008e+14+mass_l.*t6.*9.6e+14+mass_l.*z.*1.2517111896e+13+t2.*t5.*2.366016e+12+t2.*t6.*3.84e+13-t3.*t5.*1.152e+11;
    et2 = t3.*t6.*5.12e+11-t2.*z.*1.0029024e+12+t3.*z.*8.64e+9+7.5810495152267e+13;
    ik_ddelta2 = dz.*t53.*(et1+et2).*3.047761132095789e+31;
end
if nargout > 4
    t50 = cos(t49);
    t51 = sin(t49);
    ik_lt = sqrt(t9.*(t50.*1.7102875e+1+mass_l.*t50.*(1.59e+2./4.0e+2)+t8.*t50.*2.5e+1+mass_l.*t8.*t50).^2+t9.*(t51.*1.7102875e+1-tau.*1.019716212977928e-1+mass_l.*t51.*(1.59e+2./4.0e+2)+t8.*t51.*2.5e+1+mass_l.*t8.*t51-7.7e+1./1.0e+2).^2);
end
end

== matlab function DIMR_ordinary/Solution ==
  data: dz input; sol_theta1 output; mass_l input; tau input; tau_w input; z input; sol_delta2 output; sol_dtheta1 output; sol_ddelta2 output
function [sol_theta1,sol_delta2,sol_dtheta1,sol_ddelta2] = Solution(dz,mass_l,tau,tau_w,z)
%#codegen

%    This function was generated by the Symbolic Math Toolbox version 24.2.
%    20-May-2025 21:12:02

% dz = complex(dz);  % if required to enforce complex operations
% mass_l = complex(mass_l);  % if required to enforce complex operations
% tau = complex(tau);  % if required to enforce complex operations
% tau_w = complex(tau_w);  % if required to enforce complex operations
% z = complex(z);  % if required to enforce complex operations
t2 = mass_l.^2;
t3 = tau.^2;
t4 = tau_w.^2;
t5 = z.^2;
t10 = mass_l.*3.338928670752393e+104;
t15 = mass_l.*z.*4.004929483093976e+105;
t20 = z.*1.112976223584131e+107;
t35 = mass_l.*tau.*1.258123934697319e+119;
t36 = mass_l.*tau_w.*2.257868844347093e+119;
t39 = mass_l.*9.96908871603317e+119;
t46 = tau.*3.132749566128571e+121;
t47 = tau_w.*3.132749566128571e+121;
t50 = mass_l.*z.*1.329211828804423e+121;
t51 = tau.*z.*4.193746448991065e+121;
t52 = tau_w.*z.*4.193746448991065e+121;
t53 = mass_l.*tau.*z.*1.677498579596426e+120;
t54 = mass_l.*tau_w.*z.*2.148177193400137e+120;
t56 = z.*3.323029572011057e+122;
t60 = mass_l.*tau_w.*4.199100657197007e+135;
t63 = mass_l.*tau.*tau_w.*5.299370074344136e+134;
t68 = mass_l.*tau.*3.472832938331559e+136;
t70 = mass_l.*tau_w.*6.232455386016989e+136;
t71 = tau.*tau_w.*4.721738736240626e+136;
t75 = mass_l.*2.751794056482886e+137;
t76 = tau.*3.741398685562533e+137;
t77 = tau_w.*3.741398685562533e+137;
t95 = mass_l.*z.*3.669058741977181e+138;
t101 = mass_l.*tau.*z.*4.630443917775412e+137;
t102 = mass_l.*tau_w.*z.*5.929670606264586e+137;
t103 = mass_l.*6.360160640974625e+138;
t104 = tau.*8.647411896994556e+138;
t105 = tau_w.*8.647411896994557e+138;
t106 = z.*9.172646854942954e+139;
t108 = mass_l.*z.*7.628792759598937e+139;
t109 = tau.*z.*1.157610979443853e+139;
t110 = tau_w.*z.*1.157610979443853e+139;
t118 = z.*2.120053546991542e+141;
t6 = t2.*t4.*1.421335685679256e+98;
t7 = t2.*6.704631168638213e+101;
t8 = t4.*8.875461271584045e+102;
t9 = mass_l.*t4.*7.078299092538886e+100;
t12 = t2.*t4.*z.*3.790228495144683e+99;
t14 = mass_l.*t4.*z.*8.490174999599011e+101;
t17 = t2.*z.*1.78790164497019e+103;
t18 = t4.*z.*2.359433030846295e+103;
t21 = t4.*t5.*1.579261872976951e+103;
t22 = mass_l.*t4.*t5.*1.263409498381561e+102;
t23 = mass_l.*t5.*5.959672149900633e+105;
t25 = t2.*t4.*t5.*2.526818996763122e+100;
t26 = t2.*t5.*1.191934429980127e+104;
t27 = t5.*7.449590187375792e+106;
t31 = mass_l.*t4.*tau.*2.667136193497286e+115;
t32 = mass_l.*t4.*2.013986678700932e+116;
t34 = t4.*5.014860396409967e+118;
t38 = t2.*tau_w.*1.412035841411133e+117;
t40 = mass_l.*t4.*z.*2.685315571601243e+117;
t41 = mass_l.*t4.*tau.*z.*3.556181591329715e+116;
t43 = t4.*tau.*6.641213574078135e+117;
t44 = t4.*z.*6.713288929003107e+118;
t45 = -t39;
t48 = t2.*tau_w.*z.*1.882714455214844e+118;
t49 = t4.*tau.*z.*8.890453978324287e+117;
t55 = -t46;
t57 = -t51;
t58 = -t53;
t59 = t2.*t4.*2.664005273393773e+131;
t61 = mass_l.*t4.*5.559260961708241e+133;
t62 = t4.*tau.*7.931507837475262e+133;
t65 = t2.*t4.*2.707432286546221e+132;
t66 = t3.*t4.*5.004880652991975e+132;
t67 = mass_l.*t4.*tau.*7.362166928349563e+132;
t69 = -t60;
t73 = t2.*tau_w.*3.897680065467519e+134;
t79 = t2.*1.277132142550844e+136;
t80 = t3.*2.360869368120313e+136;
t81 = t4.*1.384265244900288e+136;
t82 = mass_l.*t4.*1.348310303474307e+135;
t83 = mass_l.*t4.*1.878247310908721e+135;
t85 = t4.*tau.*1.833191835437255e+135;
t86 = -t75;
t87 = -t77;
t88 = mass_l.*t4.*z.*7.412347948944321e+134;
t89 = t2.*tau_w.*z.*5.196906753956692e+135;
t90 = t4.*tau.*z.*2.454055642783188e+135;
t93 = t4.*1.445713000394586e+137;
t94 = t4.*1.690642868309707e+137;
t96 = t2.*t4.*z.*7.219819430789924e+133;
t97 = mass_l.*t4.*tau.*z.*9.81622257113275e+133;
t100 = t4.*z.*1.85308698723608e+136;
t107 = mass_l.*t4.*z.*1.617251585529328e+136;
t112 = t2.*z.*3.405685713468918e+137;
t113 = t4.*z.*4.49436767824769e+137;
t114 = -t101;
t115 = -t104;
t116 = -t108;
t117 = -t109;
t119 = t4.*t5.*3.008258096162468e+137;
t120 = mass_l.*t4.*t5.*2.406606476929975e+136;
t121 = -t118;
t122 = t2.*t4.*t5.*4.813212953859949e+134;
t123 = t2.*t5.*2.270457142312612e+138;
t124 = t5.*1.419035713945383e+141;
t125 = mass_l.*t5.*1.135228571156306e+140;
t28 = -t23;
t29 = -t26;
t30 = -t27;
t33 = -t31;
t37 = -t32;
t42 = -t38;
t64 = -t59;
t72 = -t61;
t74 = -t62;
t78 = -t67;
t84 = -t73;
t91 = -t79;
t92 = -t80;
t98 = -t83;
t99 = -t82;
t111 = -t96;
t126 = -t123;
t127 = -t124;
t128 = -t125;
t130 = 1.0./(t6-t7+t8-t9+t10-t12+t14-t15+t17+t18-t20+t21+t22+t25+t28+t29+t30-4.156994019492319e+106);
t131 = t63+t64+t66+t69+t71+t74+t76+t87+t92+t93+t98+t107+t111+t113+t119+t120+t122-1.482299731758781e+138;
t132 = t65+t91+t94+t99+t103+t107+t111+t112+t113+t116+t119+t120+t121+t122+t126+t127+t128-7.918452999352084e+140;
t135 = t68+t70+t72+t78+t81+t84+t85+t86+t88+t89+t90+t95+t97+t100+t102+t105+t106+t110+t114+t115+t117+6.852013063876662e+139;
t133 = 1.0./t132;
t136 = t135.^2;
t134 = t133.^2;
t137 = t131.*t133;
t138 = -t137;
t139 = (t134.*t136)./4.0;
t140 = t138+t139;
t141 = sqrt(abs(t140));
t142 = t2.*t4.*t141.*1.961675336397012e+115;
t143 = mass_l.*t4.*t141.*9.769208564435001e+117;
t144 = mass_l.*t141.*4.608266779901212e+121;
t145 = t2.*t141.*9.2534858131496e+118;
t146 = t4.*t141.*1.224958583045263e+120;
t147 = t2.*t4.*t141.*z.*5.231134230392032e+116;
t148 = t2.*t141.*z.*2.467596216839893e+120;
t149 = t4.*t141.*z.*3.256402854811667e+120;
t150 = t141.*5.737330543200176e+123;
t151 = mass_l.*t4.*t141.*z.*1.171782786164866e+119;
t152 = mass_l.*t141.*z.*5.527456652324976e+122;
t153 = t141.*z.*1.536088926633737e+124;
t154 = t2.*t4.*t5.*t141.*3.487422820261355e+117;
t155 = t4.*t5.*t141.*2.179639262663347e+120;
t156 = mass_l.*t4.*t5.*t141.*1.743711410130677e+119;
t157 = mass_l.*t5.*t141.*8.225320722799645e+122;
t158 = t2.*t5.*t141.*1.645064144559929e+121;
t159 = t5.*t141.*1.028165090349956e+124;
et1 = t130.*(t33+t34+t35+t36+t37+t40+t41+t42+t43+t44+t45+t47+t48+t49+t50+t52+t54+t55+t56+t57+t58-t142+t143-t144+t145-t146+t147-t148-t149+t150-t151+t152+t153-t154-t155-t156+t157+t158+t159+2.48231970544012e+122);
et2 = -7.245519476682662e-18;
et3 = t130.*(t33+t34+t35+t36+t37+t40+t41+t42+t43+t44+t45+t47+t48+t49+t50+t52+t54+t55+t56+t57+t58+t142-t143+t144-t145+t146-t147+t148+t149-t150+t151-t152-t153+t154+t155+t156-t157-t158-t159+2.48231970544012e+122);
et4 = -7.245519476682662e-18;
if tau_w >= 0
    sol_theta1 = et1.*et2;
else
    sol_theta1 = et3.*et4;
end
if nargout > 1
    sol_delta2 = z-2.41e+2./4.0e+2;
end
if nargout > 2
    sol_dtheta1 = 0.0;
end
if nargout > 3
    sol_ddelta2 = dz;
end
end

== matlab function DIMR_ordinary/simp_model_simp ==
  data: lt input; inv_cog_theta1 output; mass_l input; tau input; tau_w input; inv_cog_delta2 output; inv_cog_dtheta1 output; inv_cog_ddelta2 output
function [inv_cog_theta1,inv_cog_delta2,inv_cog_dtheta1,inv_cog_ddelta2] = simp_model_simp(lt,mass_l,tau,tau_w)
%#codegen

%    This function was generated by the Symbolic Math Toolbox version 24.2.
%    22-Apr-2025 19:32:21

% lt = complex(lt);  % if required to enforce complex operations
% mass_l = complex(mass_l);  % if required to enforce complex operations
% tau = complex(tau);  % if required to enforce complex operations
% tau_w = complex(tau_w);  % if required to enforce complex operations
t2 = lt.^2;
t3 = lt.^3;
t5 = mass_l.^2;
t6 = tau_w.^2;
t7 = mass_l+2.5e+1;
t13 = tau.*5.62949953421312e+16;
t14 = lt.*tau_w.*7.322355554724407e+34;
t15 = lt.*mass_l.*tau_w.*1.075235764276712e+33;
t4 = t2.^2;
t8 = 1.0./t7;
t9 = mass_l.*t2.*1.0e+1;
t10 = t2.*6.81e+2;
t16 = t13+4.250902933753714e+17;
t17 = t2./7.619402830239472e+32;
t18 = mass_l.*t2.*tau_w.*1.34885946680535e+34;
t20 = t2.*tau_w.*9.185732968944436e+35;
t21 = t6.*2.890329871949311e+63;
t22 = lt.*t6.*7.251709698461644e+64;
t23 = t2.*t6.*4.548554652976035e+65;
t24 = t2.*1.28908924894121e+69;
t25 = t6.*2.942683066397361e-39;
t26 = lt.*t6.*7.383061545740005e-38;
t27 = t2.*t6.*4.630943645497582e-37;
t11 = t9+t10;
t19 = 1.0./t16;
t28 = t21+t22+t23+t24;
t30 = t17+t25+t26+t27;
t12 = 1.0./t11;
t29 = 1.0./t28;
t31 = sqrt(t30);
t32 = t31.*1.526239472973816e+52;
t33 = t31.*tau.*2.021209266854921e+51;
t34 = -t32;
t35 = -t33;
t36 = t14+t15+t18+t20+t34+t35;
inv_cog_theta1 = (t12.*t36)./7.180777810073809e+34;
if nargout > 1
    et1 = t2.*7.497617546078306e+91+t6.*1.681077394732793e+86;
    et2 = lt.*t6.*4.217748764789508e+87+mass_l.*t2.*1.742574259921871e+90;
    et3 = mass_l.*t6.*3.907110730834933e+84+t2.*t6.*2.64553623447406e+88;
    et4 = t2.*tau.*9.929145675901089e+90+t6.*tau.*2.226262174908734e+85;
    et5 = t3.*tau_w.*-3.953574007462864e+91-t4.*tau_w.*4.959671083177858e+92;
    et6 = lt.*mass_l.*t6.*9.802767862150835e+85+lt.*t6.*tau.*5.585593243796743e+86;
    et7 = mass_l.*t2.*t6.*6.148677653338629e+86+mass_l.*t2.*tau.*2.307702889818632e+89;
    et8 = mass_l.*t6.*tau.*5.174213192379771e+83-mass_l.*t3.*tau_w.*1.16110837223579e+90;
    et9 = mass_l.*t4.*tau_w.*-1.456584752768827e+91+t2.*t6.*tau.*3.503501545862049e+87;
    et10 = t3.*t5.*tau_w.*-8.525024759440453e+87-t4.*t5.*tau_w.*1.069445486614411e+89;
    et11 = lt.*mass_l.*t6.*tau.*1.298187184557687e+85+mass_l.*t2.*t6.*tau.*8.14273544348634e+85;
    inv_cog_delta2 = t8.*t19.*t29.*(et1+et2+et3+et4+et5+et6+et7+et8+et9+et10+et11).*(-1.25e-4)-t8.*t12.*t19.*t29.*t36.*(t4.*4.63761e+5+mass_l.*t4.*1.362e+4+t4.*t5.*1.0e+2).*9.910645928401404e+49;
end
if nargout > 2
    inv_cog_dtheta1 = 0.0;
end
if nargout > 3
    inv_cog_ddelta2 = 0.0;
end
end

== matlab function DIMR_ordinary/Plant model/MBD model/MATLAB Function ==
  data: u input; rotx output; roty output; rotz output
function [rotx,roty,rotz] = calculate_rot2eul(u)

rot  = rotm2eul(u);
rotx  = rot(1);
roty  = rot(2);
rotz  = rot(3);

== matlab function DIMR_ordinary/Plant model/MATLAB Function ==
  data: u input; rotx output; roty output; rotz output
function [rotx,roty,rotz] = calculate_rot2eul(u)

rot  = rotm2eul(u);
rotx  = rot(1);
roty  = rot(2);
rotz  = rot(3);

== matlab function DIMR_ordinary/Calc_states/Calc_XY ==
  data: v input; X output; phi input; Xp input; Yp input; Y output
function [X,Y] = fcn(v,phi,Xp,Yp)

X = Xp+v*cos(phi);
Y = Yp+v*sin(phi);

end
